simulink model "KF_feedback"  (R2019b)
settings: Solver=VariableStepAuto  StartTime=0.0  StopTime=10.0  RelTol=1e-3
values from neighbouring files (symbols this model uses):
  data = e_h.load_data    [potentiometer_recover.m]
  experiment = merge( experiment, experiment2 )    [blackbox_est.m]
undefined symbols (not defined in the file or in its folder): K_v, K_x
libraries: simulink x2
settings Model: Creator=giacomo  LastModifiedBy=giacomo

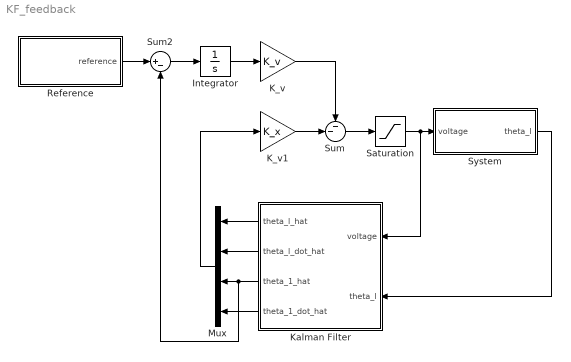
== system KF_feedback ==
  Integrator : Integrator
  K_v : Gain  Gain=K_v
  K_v1 : Gain  Gain=K_x
  Kalman Filter : Subsystem
  Mux : Mux
  Reference : Subsystem
  Saturation : Saturate
  Sum : Sum  Inputs=--|
  Sum2 : Sum  Inputs=|+-
  System : Subsystem
  wires:
  Kalman Filter/3(theta_1_hat) -> Sum2/2, Mux/3
  Reference/1(reference) -> Sum2/1
  Mux/1 -> K_v1/1
  Integrator/1 -> K_v/1
  Sum2/1 -> Integrator/1
  K_v/1 -> Sum/1
  K_v1/1 -> Sum/2
  Kalman Filter/1(theta_l_hat) -> Mux/1
  Kalman Filter/2(theta_l_dot_hat) -> Mux/2
  Kalman Filter/4(theta_1_dot_hat) -> Mux/4
  Sum/1 -> Saturation/1
  Saturation/1 -> Kalman Filter/1(voltage), System/1(voltage)
  System/1(theta_l) -> Kalman Filter/2(theta_l)

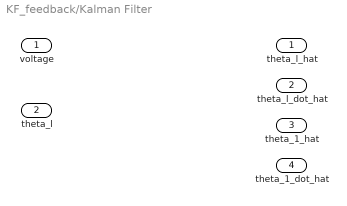
== system KF_feedback/Kalman Filter ==
  voltage : Inport
  theta_l : Inport  Port=2
  theta_l_hat : Outport
  theta_l_dot_hat : Outport  Port=2
  theta_1_hat : Outport  Port=3
  theta_1_dot_hat : Outport  Port=4

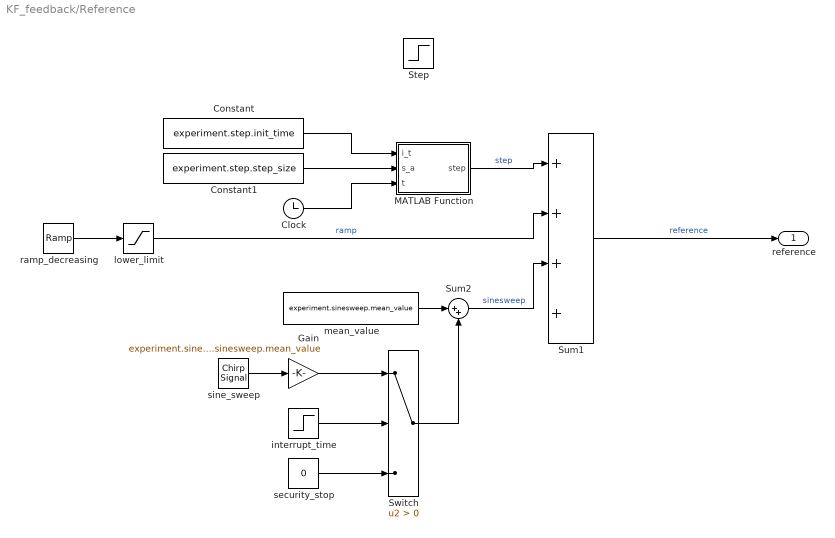
== system KF_feedback/Reference ==
  Clock : Clock
  Constant : Constant  Value=experiment.step.init_time
  Constant1 : Constant  Value=experiment.step.step_size
  Gain : Gain  Gain=experiment.sinesweep.v_max-experiment.sinesweep.mean_value
  MATLAB Function : MATLAB Function  TreatAsAtomicUnit=on
  Step : Step  Before=-data.motor_pos_0  After=0  SampleTime=0
  Sum1 : Sum  Inputs=++++
  Sum2 : Sum  Inputs=|++
  Switch : Switch  Criteria=u2 > Threshold
  interrupt_time : Step  Time=experiment.sinesweep.target_time  Before=1  After=-1  SampleTime=0
  lower_limit : Saturate  UpperLimit=max( experiment.ramp.init_value, experiment.ramp.final_value )  LowerLimit=min( experiment.ramp.init_value, experiment.ramp.final_value )
  mean_value : Constant  Value=experiment.sinesweep.mean_value
  ramp_decreasing : simulink/Sources/Ramp  slope=experiment.ramp.ramp_pend  start=experiment.ramp.init_time  InitialOutput=experiment.ramp.init_value
  security_stop : Constant  Value=0
  sine_sweep : simulink/Sources/Chirp Signal  f1=experiment.sinesweep.init_freq  T=experiment.sinesweep.target_time  f2=experiment.sinesweep.final_freq
  reference : Outport
  wires:
  mean_value/1 -> Sum2/1
  lower_limit/1 -> Sum1/2  "ramp"
  Switch/1 -> Sum2/2
  interrupt_time/1 -> Switch/2
  Sum2/1 -> Sum1/3  "sinesweep"
  Sum1/1 -> reference/1  "reference"
  security_stop/1 -> Switch/3
  ramp_decreasing/1 -> lower_limit/1
  Gain/1 -> Switch/1
  sine_sweep/1 -> Gain/1
  Clock/1 -> MATLAB Function/3(t)
  Constant/1 -> MATLAB Function/1(i_t)
  Constant1/1 -> MATLAB Function/2(s_a)
  MATLAB Function/1(step) -> Sum1/1  "step"

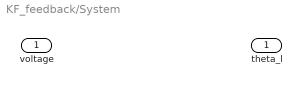
== system KF_feedback/System ==
  voltage : Inport
  theta_l : Outport

== matlab function KF_feedback/Reference/MATLAB Function ==
  data: i_t input; step output; s_a input; t input
function step = multistep(i_t, s_a, t)

% it is assumed i_t is sorted!

% find the first time step that is greater than actual time. 
step = 0;
for idx = 1:length(i_t) 
    if i_t(idx) <= t
        step = s_a(idx);
    end
end
